simulink model "datamngtworkflow"  (Simulink 6.4)
settings: Solver=FixedStepDiscrete  StartTime=0.0  StopTime=10.0  FixedStep=1  RelTol=1e-3
undefined symbols (not defined in the file or in its folder): K1, LOWER, T1Break, T1Data, T2Data, UPPER
settings Model: Creator=The MathWorks Inc.  LastModifiedBy=t_fukuda  CovMetricSettings=d  ExtModeAutoUpdateStatusClock=off  ProdHWDeviceType=Hitachi SH-2
settings DataIOCC: SaveOutput=off  SignalLogging=off  SaveTime=off  SignalLoggingName=sigsOut
settings OptimizationCC: InlineParams=on  InlineInvariantSignals=on  EnforceIntegerDowncast=off  StateBitsets=on  DataBitsets=on  UseTempVars=on  ZeroExternalMemoryAtStartup=off  ZeroInternalMemoryAtStartup=off  InitFltsAndDblsToZero=off  NoFixptDivByZeroProtection=on  OptimizeModelRefInitCode=on  LifeSpan=1
settings DebuggingCC: CheckExecutionContextPreStartOutputMsg=on  CheckExecutionContextRuntimeOutputMsg=on  SignalResolutionControl=UseLocalSettings  SolverPrmCheckMsg=none  ParameterDowncastMsg=warning  ParameterOverflowMsg=warning
settings HardwareCC: ProdIntDivRoundTo=Floor  ProdEndianess=BigEndian  ProdHWDeviceType=Hitachi SH-2
settings RTWCC: SystemTargetFile=ert.tlc  TLCOptions=-p0  GenCodeOnly=on  TemplateMakefile=ert_default_tmf  Description=RTW Embedded Coder (no auto configuration)  RTWVerbose=off  ProcessScript=ert_make_rtw_hook
settings CodeAppCC: IgnoreCustomStorageClasses=off  SimulinkDataObjDesc=on  PrefixModelToSubsysFcnNames=off  CustomCommentsFcn=custom_comments_example.m  EnableCustomComments=on
settings ERTTargetCC: TargetFcnLib=ansi_tfl_tmw.mat  GenFloatMathFcnCalls=ANSI_C  IncludeMdlTerminateFcn=off  SuppressErrorStatus=on  IncludeERTFirstTime=on  SupportAbsoluteTime=off  SupportNonFinite=off  SupportComplex=off  InlinedParameterPlacement=NonHierarchical  ERTCustomFileTemplate=example_file_process.tlc  InitialValueSource=DataObject  ModuleNamingRule=SameAsModel  EnableUserReplacementTypes=on
settings MATStruct: int32=s32  int16=s16  int8=s08  uint32=u32  uint16=u16  uint8=u08  boolean=bool  int=sint  uint=uint

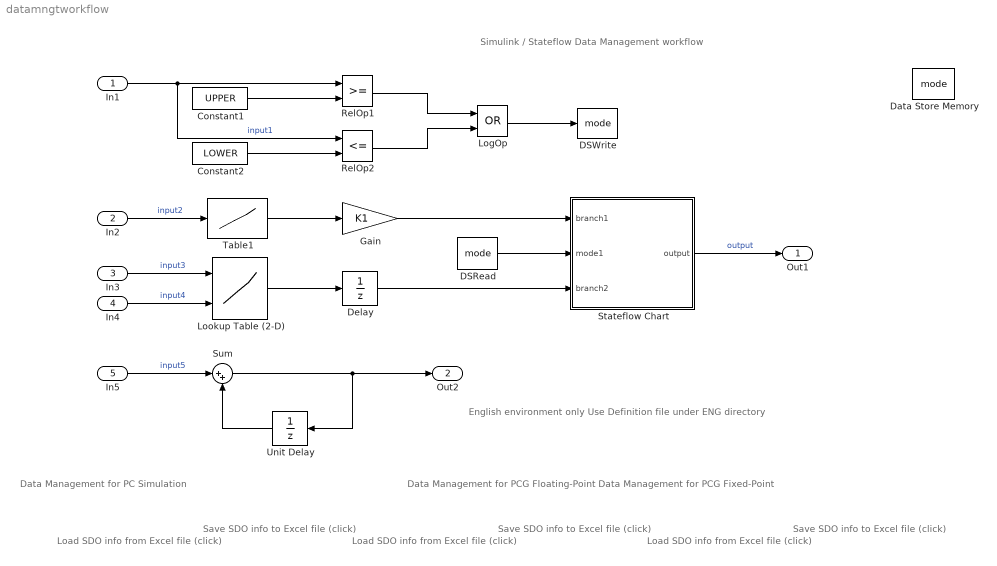
== system datamngtworkflow ==
  note: Simulink / Stateflow Data Management workflow
  note: Data Management for PC Simulation
  note: Data Management for PCG Floating-Point
  note: Data Management for PCG Fixed-Point
  note: Load SDO info
      | from Excel file
      | (click)
  note: Save SDO info
      | to Excel file
      | (click)
  note: Load SDO info
      | from Excel file
      | (click)
  note: Save SDO info
      | to Excel file
      | (click)
  note: Load SDO info
      | from Excel file
      | (click)
  note: Save SDO info
      | to Excel file
      | (click)
  note: English environment only
      | Use Definition file under ENG directory
  In1 : Inport  PortDimensions=1  OutDataType=input1.DataType
  In2 : Inport  Port=2  PortDimensions=1  OutDataType=input2.DataType
  In3 : Inport  Port=3  PortDimensions=1  OutDataType=input3.DataType
  In4 : Inport  Port=4  PortDimensions=1  OutDataType=input4.DataType
  In5 : Inport  Port=5  PortDimensions=2  OutDataType=input5.DataType
  Constant1 : Constant  Value=UPPER  OutDataType=sfix(16)  ConRadixGroup=Use specified scaling  OutScaling=2^0  SampleTime=Inf  FramePeriod=inf
  Constant2 : Constant  Value=LOWER  OutDataType=sfix(16)  ConRadixGroup=Use specified scaling  OutScaling=2^0  SampleTime=Inf  FramePeriod=inf
  DSRead : DataStoreRead  DataStoreName=mode  SampleTime=1
  DSWrite : DataStoreWrite  DataStoreName=mode  SampleTime=-1
  Data Store Memory : DataStoreMemory  DataStoreName=mode  InitialValue=0  StateMustResolveToSignalObject=on
  Delay : UnitDelay  SampleTime=-1  StateIdentifier=X  StateMustResolveToSignalObject=on
  Gain : Gain  Gain=K1
  LogOp : Logic  Operator=OR  OutDataTypeMode=Boolean
  Lookup Table (2-D) : Lookup2D  RowIndex=T2Break  ColumnIndex=T2Break  OutputValues=T2Data  LookUpMeth=Interpolation-Use End Values
  RelOp1 : RelationalOperator  InputSameDT=on
  RelOp2 : RelationalOperator  Operator=<=  InputSameDT=on
  Stateflow Chart : Stateflow chart
  Sum : Sum  Inputs=|++
  Table1 : Lookup  InputValues=T1Break  OutputValues=T1Data  LookUpMeth=Interpolation-Use End Values
  Unit Delay : UnitDelay  Orientation=left  X0=[0 0]  SampleTime=-1  StateIdentifier=state1  StateMustResolveToSignalObject=on
  Out1 : Outport  PortDimensions=1  OutDataType=output.DataType
  Out2 : Outport  Port=2  OutDataType=output.DataType
  wires:
  RelOp1/1 -> LogOp/1
  RelOp2/1 -> LogOp/2
  Constant2/1 -> RelOp2/2
  In2/1 -> Table1/1  "input2"
  Gain/1 -> Stateflow Chart/1(branch1)
  Table1/1 -> Gain/1
  Lookup Table (2-D)/1 -> Delay/1
  Constant1/1 -> RelOp1/2
  In1/1 -> RelOp2/1, RelOp1/1  "input1"
  In3/1 -> Lookup Table (2-D)/1  "input3"
  In4/1 -> Lookup Table (2-D)/2  "input4"
  Stateflow Chart/1(output) -> Out1/1  "output"
  Delay/1 -> Stateflow Chart/3(branch2)
  LogOp/1 -> DSWrite/1
  DSRead/1 -> Stateflow Chart/2(mode1)
  In5/1 -> Sum/1  "input5"
  Unit Delay/1 -> Sum/2
  Sum/1 -> Out2/1, Unit Delay/1

== stateflow chart Stateflow Chart ==
  note: This chart is acting as an if-else condition,
      |     with the result multiplied by K2.
      | Using a Simulink switch (or if-action) and gain block,
      |     results in virtually identical code.
  (junction 7) -> (junction 4) : {output = branch1;}
  (junction 4) -> (junction 6) : {output *= K2;}
  (junction 5) -> (junction 4) [order 2] : {output = branch2;}
  (default) -> (junction 5)
  (junction 5) -> (junction 7) [order 1] : [mode1]
  data: branch1 input inherited; mode1 input boolean size=1; branch2 input inherited; output output type(branch1) size=size(branch1); K2 parameter inherited size=[1 1]
  data branch1 settings: units=Nm
  data branch2 settings: units=Nm
  data output settings: units=V
  data K2 settings: units=V/Nm
